simulink model "clark_plark"  (R2019b)
settings: Solver=VariableStepAuto  StartTime=0.0  StopTime=0.05  MaxStep=1e-4  RelTol=1e-3
settings Model: Creator=kissd  LastModifiedBy=kissd

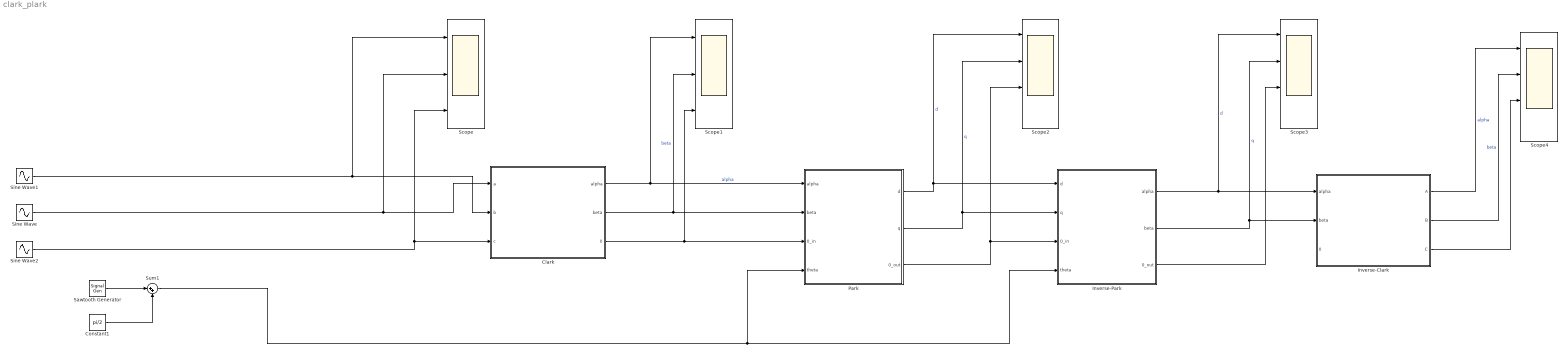
== system clark_plark ==
  Clark : Subsystem
  Constant1 : Constant  Value=pi/2
  Inverse-Clark : Subsystem
  Inverse-Park : Subsystem
  Park : Subsystem
  Sawtooth Generator : SignalGenerator  WaveForm=sawtooth  Amplitude=-pi  Frequency=100*2*pi  Units=rad/sec
  Scope : Scope  NumInputPorts=3
  Scope1 : Scope  NumInputPorts=3
  Scope2 : Scope  NumInputPorts=4
  Scope3 : Scope  NumInputPorts=4
  Scope4 : Scope  NumInputPorts=4
  Sine Wave : Sin  Amplitude=200  Frequency=2*pi*100  SampleTime=0
  Sine Wave1 : Sin  Amplitude=200  Frequency=2*pi*100  Phase=-2*pi/3  SampleTime=0
  Sine Wave2 : Sin  Amplitude=200  Frequency=2*pi*100  Phase=+2*pi/3  SampleTime=0
  Sum1 : Sum  Inputs=|++
  wires:
  Sine Wave1/1 -> Clark/2(b), Scope/1
  Sine Wave2/1 -> Scope/3, Clark/3(c)
  Sine Wave/1 -> Clark/1(a), Scope/2
  Clark/1(alpha) -> Scope1/1, Park/1(alpha)  "alpha"
  Clark/2(beta) -> Scope1/2, Park/2(beta)  "beta"
  Clark/3(0) -> Scope1/3, Park/3(0_in)
  Park/1(d) -> Inverse-Park/1(d), Scope2/1  "d"
  Park/2(q) -> Scope2/2, Inverse-Park/2(q)  "q"
  Park/3(0_out) -> Inverse-Park/3(0_in), Scope2/3
  Constant1/1 -> Sum1/2
  Sawtooth Generator/1 -> Sum1/1
  Sum1/1 -> Inverse-Park/4(theta), Park/4(theta)
  Inverse-Park/1(alpha) -> Scope3/1, Inverse-Clark/1(alpha)  "d"
  Inverse-Park/2(beta) -> Inverse-Clark/2(beta), Scope3/2  "q"
  Inverse-Park/3(0_out) -> Scope3/3
  Inverse-Clark/1(A) -> Scope4/1  "alpha"
  Inverse-Clark/2(B) -> Scope4/2  "beta"
  Inverse-Clark/3(C) -> Scope4/3

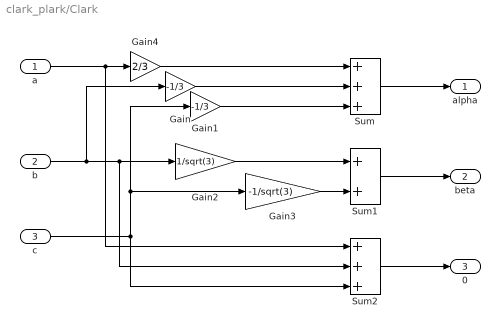
== system clark_plark/Clark ==
  a : Inport
  b : Inport  Port=2
  c : Inport  Port=3
  Gain : Gain  Gain=-1/3
  Gain1 : Gain  Gain=-1/3
  Gain2 : Gain  Gain=1/sqrt(3)
  Gain3 : Gain  Gain=-1/sqrt(3)
  Gain4 : Gain  Gain=2/3
  Sum : Sum  Inputs=+++
  Sum1 : Sum
  Sum2 : Sum  Inputs=+++
  alpha : Outport
  beta : Outport  Port=2
  0 : Outport  Port=3
  wires:
  Sum/1 -> alpha/1
  a/1 -> Sum2/1, Gain4/1
  Gain/1 -> Sum/2
  Gain1/1 -> Sum/3
  b/1 -> Sum2/2, Gain2/1, Gain/1
  c/1 -> Gain3/1, Gain1/1, Sum2/3
  Sum1/1 -> beta/1
  Gain2/1 -> Sum1/1
  Gain3/1 -> Sum1/2
  Sum2/1 -> 0/1
  Gain4/1 -> Sum/1

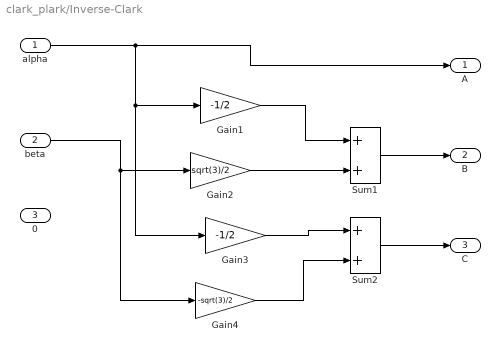
== system clark_plark/Inverse-Clark ==
  alpha : Inport
  beta : Inport  Port=2
  0 : Inport  Port=3
  Gain1 : Gain  Gain=-1/2
  Gain2 : Gain  Gain=sqrt(3)/2
  Gain3 : Gain  Gain=-1/2
  Gain4 : Gain  Gain=-sqrt(3)/2
  Sum1 : Sum
  Sum2 : Sum
  A : Outport
  B : Outport  Port=2
  C : Outport  Port=3
  wires:
  alpha/1 -> Gain3/1, Gain1/1, A/1
  Sum1/1 -> B/1
  Gain2/1 -> Sum1/2
  Sum2/1 -> C/1
  Gain1/1 -> Sum1/1
  beta/1 -> Gain4/1, Gain2/1
  Gain3/1 -> Sum2/1
  Gain4/1 -> Sum2/2

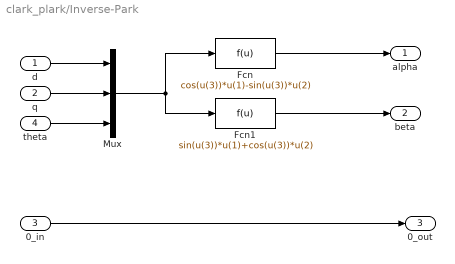
== system clark_plark/Inverse-Park ==
  d : Inport
  q : Inport  Port=2
  0_in : Inport  Port=3
  theta : Inport  Port=4
  Fcn : Fcn  Expr=cos(u(3))*u(1)-sin(u(3))*u(2)
  Fcn1 : Fcn  Expr=sin(u(3))*u(1)+cos(u(3))*u(2)
  Mux : Mux  Inputs=3
  alpha : Outport
  beta : Outport  Port=2
  0_out : Outport  Port=3
  wires:
  0_in/1 -> 0_out/1
  Fcn/1 -> alpha/1
  Mux/1 -> Fcn1/1, Fcn/1
  q/1 -> Mux/2
  d/1 -> Mux/1
  theta/1 -> Mux/3
  Fcn1/1 -> beta/1

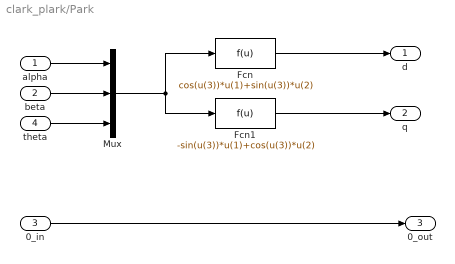
== system clark_plark/Park ==
  alpha : Inport
  beta : Inport  Port=2
  0_in : Inport  Port=3
  theta : Inport  Port=4
  Fcn : Fcn  Expr=cos(u(3))*u(1)+sin(u(3))*u(2)
  Fcn1 : Fcn  Expr=-sin(u(3))*u(1)+cos(u(3))*u(2)
  Mux : Mux  Inputs=3
  d : Outport
  q : Outport  Port=2
  0_out : Outport  Port=3
  wires:
  0_in/1 -> 0_out/1
  Fcn/1 -> d/1
  Mux/1 -> Fcn1/1, Fcn/1
  beta/1 -> Mux/2
  alpha/1 -> Mux/1
  theta/1 -> Mux/3
  Fcn1/1 -> q/1
